simulink model "sim6"  (R2015b)
settings: Solver=VariableStepAuto  StartTime=0.0  StopTime=10.0  RelTol=1e-3
values from neighbouring files (symbols this model uses):
  beta = 0.001    [Lab3.m]    (also in calc_erro_l1.m; calc_erro_l2.m)
  dteta_inicial = 0    [Lab3.m]    (also in calc_erro_l1.m; calc_erro_l2.m)
  g = 9.8    [Lab3.m]    (also in calc_erro_l1.m; calc_erro_l2.m)
  J = (m*l^2)+(M/3)*L^2    (= 0.00626971061233)    [Lab3.m]    (also in fcn.m = (m*l^2)+(M/3)*L^2)
  k = 0.35    [Lab3.m]    (also in calc_erro_l1.m; calc_erro_l2.m; calc_media_BPM.m = 2)
  l = 0.2289    [Lab3.m]    (also in calc_erro_l1.m = x; calc_erro_l2.m = x; parametros_estimados.m = l_set(ind_c))
  L = 0.25    [Lab3.m]    (also in calc_erro_l1.m; calc_erro_l2.m)
  m = 0.0799    [Lab3.m]    (also in calc_erro_l1.m; calc_erro_l2.m; parametros_estimados.m = m_set(ind_r))
  M = 0.1    [Lab3.m]    (also in calc_erro_l1.m; calc_erro_l2.m)
  teta_inicial = pi/4    (= 0.785398163397)    [Lab3.m]    (also in calc_erro_l1.m; calc_erro_l2.m)
settings Model: Creator=Alice  LastModifiedBy=Alice

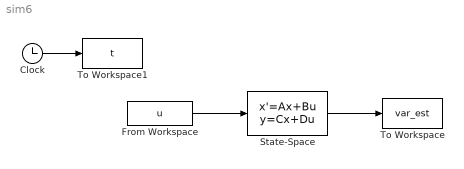
== system sim6 ==
  Clock : Clock
  From Workspace : FromWorkspace  VariableName=u  SampleTime=0.01
  State-Space : StateSpace  A=[0 1; ((g*(m*l+(1/2)*M*L)-k)/J) -(beta/J)]  B=[0; 1/J]  C=[1 0; 0 1]  D=[0; 0]  X0=[teta_inicial; dteta_inicial]
  To Workspace : ToWorkspace  VariableName=var_est  SampleTime=0.01
  To Workspace1 : ToWorkspace  VariableName=t  SampleTime=0.01
  wires:
  Clock/1 -> To Workspace1/1
  From Workspace/1 -> State-Space/1
  State-Space/1 -> To Workspace/1
